simulink model "yaw_control"  (R2015a)
settings: Solver=ode45  StartTime=0.0  StopTime=300  FixedStep=0.001  RelTol=1e-6
InitFcn:
  | parameters
values from neighbouring files (symbols this model uses):
  data = load_filters(path)    [filtering.m]    (also in load_filters.m = dlmread(path, ' '); load_measures.m = dlmread(path, ' '); plot_data.m; yaw_mode.m = load_measures(path))
settings Model: Creator=GSavaia  LastModifiedBy=GSavaia

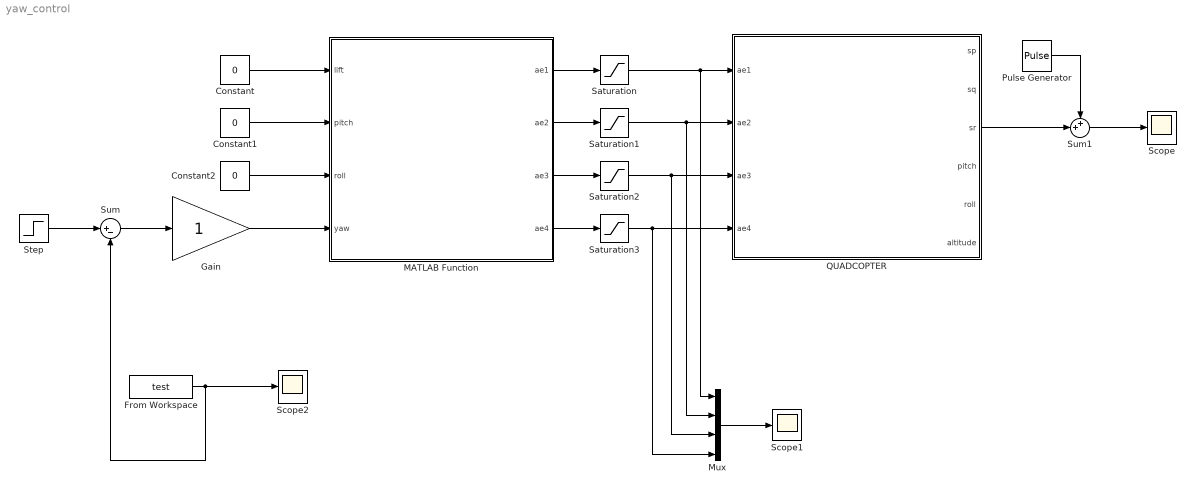
== system yaw_control ==
  Constant : Constant  Value=0
  Constant1 : Constant  Value=0
  Constant2 : Constant  Value=0
  From Workspace : FromWorkspace  VariableName=test  SampleTime=0
  Gain : Gain
  MATLAB Function : MATLAB Function  TreatAsAtomicUnit=on
  Mux : Mux
  Pulse Generator : DiscretePulseGenerator  PulseType=Time based  Amplitude=10  Period=3  PulseWidth=0.5  PhaseDelay=1
  QUADCOPTER : Subsystem
  Saturation : Saturate  UpperLimit=1023  LowerLimit=0
  Saturation1 : Saturate  UpperLimit=1023
  Saturation2 : Saturate  UpperLimit=1023
  Saturation3 : Saturate  UpperLimit=1023
  Scope : Scope
  Scope1 : Scope
  Scope2 : Scope
      settings: SaveName=ScopeData2
  Step : Step  Time=0  After=mean(data.sr)  SampleTime=0
  Sum : Sum  Inputs=|+-
  Sum1 : Sum  Inputs=++|
  wires:
  Gain/1 -> MATLAB Function/4(yaw)
  Sum/1 -> Gain/1
  Step/1 -> Sum/1
  Constant/1 -> MATLAB Function/1(lift)
  Constant1/1 -> MATLAB Function/2(pitch)
  Constant2/1 -> MATLAB Function/3(roll)
  QUADCOPTER/3(sr) -> Sum1/2
  Sum1/1 -> Scope/1
  Pulse Generator/1 -> Sum1/1
  Mux/1 -> Scope1/1
  MATLAB Function/1(ae1) -> Saturation/1
  MATLAB Function/2(ae2) -> Saturation1/1
  Saturation1/1 -> Mux/2, QUADCOPTER/2(ae2)
  MATLAB Function/3(ae3) -> Saturation2/1
  Saturation2/1 -> Mux/3, QUADCOPTER/3(ae3)
  MATLAB Function/4(ae4) -> Saturation3/1
  Saturation3/1 -> Mux/4, QUADCOPTER/4(ae4)
  Saturation/1 -> Mux/1, QUADCOPTER/1(ae1)
  From Workspace/1 -> Scope2/1, Sum/2

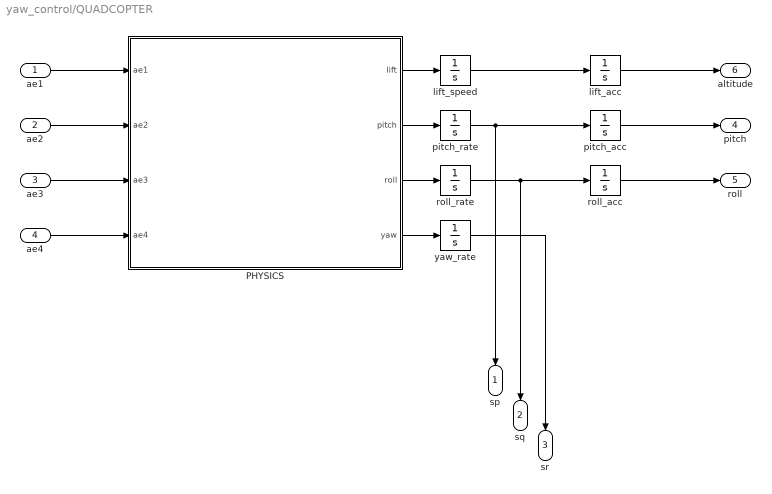
== system yaw_control/QUADCOPTER ==
  ae1 : Inport
  ae2 : Inport  Port=2
  ae3 : Inport  Port=3
  ae4 : Inport  Port=4
  PHYSICS : MATLAB Function  TreatAsAtomicUnit=on
  lift_acc : Integrator
  lift_speed : Integrator
  pitch_acc : Integrator
  pitch_rate : Integrator
  roll_acc : Integrator
  roll_rate : Integrator
  yaw_rate : Integrator
  sp : Outport
  sq : Outport  Port=2
  sr : Outport  Port=3
  pitch : Outport  Port=4
  roll : Outport  Port=5
  altitude : Outport  Port=6
  wires:
  roll_acc/1 -> roll/1
  ae4/1 -> PHYSICS/4(ae4)
  pitch_rate/1 -> pitch_acc/1, sp/1
  PHYSICS/1(lift) -> lift_speed/1
  PHYSICS/4(yaw) -> yaw_rate/1
  PHYSICS/2(pitch) -> pitch_rate/1
  PHYSICS/3(roll) -> roll_rate/1
  lift_speed/1 -> lift_acc/1
  pitch_acc/1 -> pitch/1
  lift_acc/1 -> altitude/1
  ae3/1 -> PHYSICS/3(ae3)
  ae1/1 -> PHYSICS/1(ae1)
  ae2/1 -> PHYSICS/2(ae2)
  roll_rate/1 -> roll_acc/1, sq/1
  yaw_rate/1 -> sr/1

== matlab function yaw_control/MATLAB Function ==
  data: lift input; ae1 output; pitch input; roll input; yaw input; ae2 output; ae3 output; ae4 output
function [ae1, ae2, ae3, ae4] = interface(lift, pitch, roll, yaw)

% PARAMETERS
scale_lift = -16400;
scale_pitch = 8240;
scale_roll = 8240;
scale_yaw = 16400;

scales = diag( [scale_pitch, scale_roll, scale_yaw, scale_lift] );
coeff = [+2 +0 -1 -1; ...
         +0 -2 +1 -1; ...
         -2 +0 -1 -1; ...
         +0 +2 +1 -1];
motors = 1/4.*coeff*scales*[pitch;roll;yaw;lift];

motors( motors < 0 ) = 0;

motors = round(motors);

ae1 = sqrt( motors(1) );
ae2 = sqrt( motors(2) );
ae3 = sqrt( motors(3) );
ae4 = sqrt( motors(4) );

end

== matlab function yaw_control/QUADCOPTER/PHYSICS ==
  data: ae1 input; lift output; ae2 input; ae3 input; ae4 input; pitch output; roll output; yaw output
function [lift, pitch, roll, yaw] = motor_to_forces(ae1, ae2, ae3, ae4)

% PARAMETERS
scale_lift = 16400;
scale_pitch = 8240;
scale_roll = 8240;
scale_yaw = 16400;

lift    = 1/scale_lift*( ae1^2 + ae2^2 + ae3^2 + ae4^2 );
pitch   = 1/scale_pitch*( ae4^2 - ae2^2 );
roll    = 1/scale_roll*( ae1^2 - ae3^2 );
yaw     = 1/scale_yaw*( ae2^2 + ae4^2 - ae1^2 - ae3^2 );

end
